simulink model "passive_new_wave_architecture_variable - Copy"  (R2021b)
settings: Solver=VariableStepAuto  StartTime=0.0  StopTime=20  RelTol=1e-5
values from neighbouring files (symbols this model uses):
  a1 = 1    [new_parameters.m]    (also in old.m; paper.m = 1.9; teleop_parameters_variable.m = 1.1)
  a2 = 1    [new_parameters.m]    (also in old.m; paper.m = 2.3; teleop_parameters_variable.m = 1.0101)
  b = 1    [new_parameters.m]    (also in old.m = 8.5; paper.m = 2.5; teleop_parameters_variable.m = 2.17; wave_s.m = block.InputPort(3).Data)
  B = 1.1    [new_parameters.m]    (also in obs_m.m = block.InputPort(4).Data; obs_s.m = block.InputPort(4).Data; old.m = 13; paper.m = 2)
  Be = 5    [new_parameters.m]    (also in old.m; paper.m; teleop_parameters_variable.m)
  beta = 1e-2    (= 0.01)    [new_parameters.m]    (also in old.m = 1.19e-07; paper.m = 2; teleop_parameters_variable.m = 0.0001)
  beta_m = 2*pi*Fc_vel*Ts    (= 0.0628318530718)    [new_parameters.m]    (also in old.m; paper.m; teleop_parameters_variable.m)
  beta_s = 2*pi*Fc_vel*Ts    (= 0.0628318530718)    [new_parameters.m]    (also in old.m; paper.m; teleop_parameters_variable.m)
  Bh = 0.02    [new_parameters.m]    (also in old.m; paper.m; teleop_parameters_variable.m)
  d_m2s = 1    [new_parameters.m]    (also in old.m = 2; paper.m = 2; teleop_parameters_variable.m = 2)
  delta = 1    [new_parameters.m]    (also in old.m; paper.m; teleop_parameters_variable.m = 100)
  eQ_m = 2*pi/4096    (= 0.00153398078789)    [new_parameters.m]    (also in old.m; paper.m; teleop_parameters_variable.m)
  eQ_s = 2*pi/4096    (= 0.00153398078789)    [new_parameters.m]    (also in old.m; paper.m; teleop_parameters_variable.m)
  Fc_h = 5    [new_parameters.m]    (also in old.m; paper.m; teleop_parameters_variable.m)
  Filter = 1    [old.m]
  Jh = 0.02    [new_parameters.m]    (also in old.m; paper.m; teleop_parameters_variable.m)
  k_m = 19.34    [new_parameters.m]    (also in old.m; paper.m; teleop_parameters_variable.m)
  k_s = 19.34    [new_parameters.m]    (also in old.m; paper.m; teleop_parameters_variable.m)
  ka = 0.001    [new_parameters.m]    (also in old.m = 0.0109; paper.m = 0.9; teleop_parameters_variable.m = 1)
  kb = 0.001    [new_parameters.m]    (also in old.m = 0.0089999; paper.m = 0.9; teleop_parameters_variable.m = 0.1)
  Kc2v_m = 4.5    [new_parameters.m]    (also in old.m; paper.m; teleop_parameters_variable.m)
  Kc2v_s = 4.5    [new_parameters.m]    (also in old.m; paper.m; teleop_parameters_variable.m)
  Kd_h = 0.5    [new_parameters.m]    (also in old.m; paper.m; teleop_parameters_variable.m)
  Kd_m = 0.5    [new_parameters.m]    (also in old.m; paper.m; teleop_parameters_variable.m)
  Kd_s = 0.5    [new_parameters.m]    (also in old.m; paper.m; teleop_parameters_variable.m)
  Ke = 10    [new_parameters.m]    (also in old.m; paper.m; teleop_parameters_variable.m = 100)
  Kp_h = 1.2    [new_parameters.m]    (also in old.m; paper.m; teleop_parameters_variable.m)
  Kp_m = 1    [new_parameters.m]    (also in old.m; paper.m; teleop_parameters_variable.m)
  Kp_s = 1    [new_parameters.m]    (also in old.m; paper.m; teleop_parameters_variable.m)
  Kt2c_m = 1.182    [new_parameters.m]    (also in old.m; paper.m; teleop_parameters_variable.m)
  Kt2c_s = 1.182    [new_parameters.m]    (also in old.m; paper.m; teleop_parameters_variable.m)
  lArm_m = 0.1    [new_parameters.m]    (also in old.m; paper.m; teleop_parameters_variable.m)
  lArm_s = 0.1    [new_parameters.m]    (also in old.m; paper.m; teleop_parameters_variable.m)
  M = 2    [new_parameters.m]    (also in obs_m.m = block.InputPort(5).Data; obs_s.m = block.InputPort(5).Data; old.m = 1; paper.m = 1)
  qe = 0.5    [new_parameters.m]    (also in old.m; paper.m; teleop_parameters_variable.m = 10)
  tau_m = 1.217    [new_parameters.m]    (also in old.m; paper.m; teleop_parameters_variable.m)
  tau_s = 1.217    [new_parameters.m]    (also in old.m; paper.m; teleop_parameters_variable.m)
  Ts = 0.001    [new_parameters.m]    (also in old.m; paper.m; teleop_parameters_variable.m)
libraries: simulink x2
settings Model: DataTypeOverride=Off  Creator=riccardo  LastModifiedBy=luigi
settings DebuggingCC: IgnoredZcDiagnostic=none  SFMachineParentedDataDiag=warning

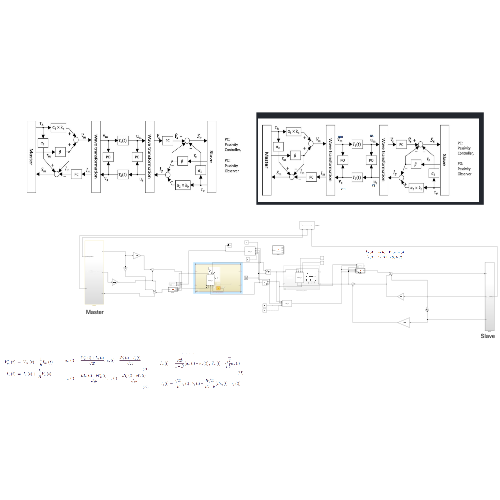
[thumbnail: Simulink's stored preview of the top-level diagram]
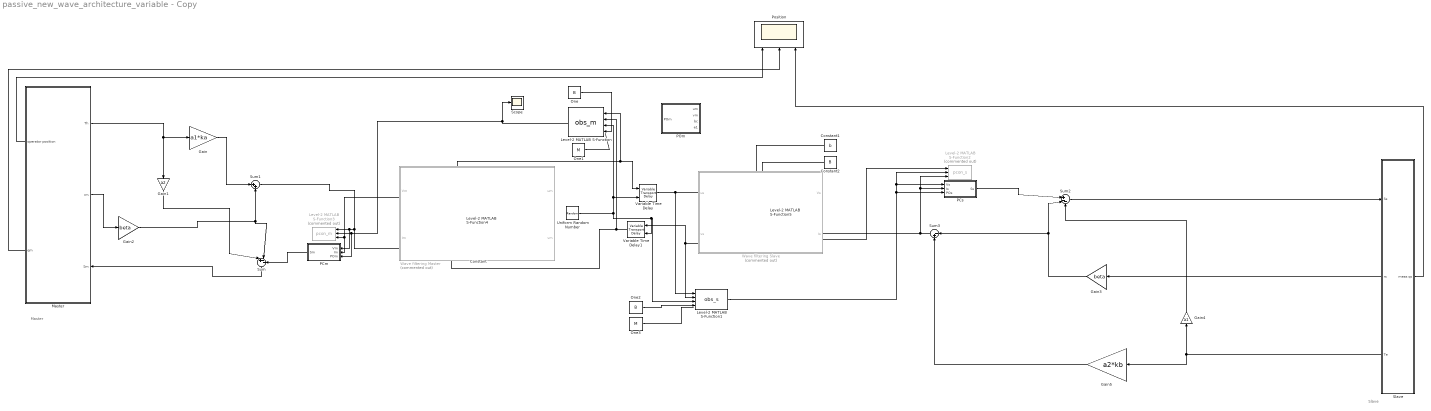
== system passive_new_wave_architecture_variable - Copy ==
  note: Slave
  note: Master
  Constant : Constant  Value=b
  Constant1 : Constant  Value=b
  Constant2 : Constant  Value=B
  Gain : Gain  Gain=a1*ka
  Gain1 : Gain  Gain=a2
  Gain2 : Gain  Gain=beta
  Gain3 : Gain  Gain=beta
  Gain4 : Gain  Gain=a1
  Gain5 : Gain  Gain=a2*kb
  Level-2 MATLAB S-Function : M-S-Function  FunctionName=obs_m
  Level-2 MATLAB S-Function1 : M-S-Function  FunctionName=obs_s
  Level-2 MATLAB S-Function2 : M-S-Function  Commented=on  FunctionName=pcon_s
  Level-2 MATLAB S-Function3 : M-S-Function  Commented=on  FunctionName=pcon_m
  Level-2 MATLAB S-Function4 : M-S-Function  FunctionName=wave_m
  Level-2 MATLAB S-Function5 : M-S-Function  FunctionName=wave_s
  Master : Subsystem
      settings: PortSchema="{\"entries\":[{\"content\":{\"sides\":[{\"content\":{\"connectorIds\":[\"Out3\",\"Out4\"]},\"type\":\"ConnectorPlacement.EquallySpacedRectSide\",\"uuid\":\"88a440f3-3c17-4ecd-8a7c-55e312326b6c\"},{\"content\":{\"connectorIds\":[\"Out1\",\"Out2\",\"In1\"],\"side\":\"RIGHT\"},\"type\":\"ConnectorPlacement.EquallySpacedRectSide\",\"uuid\":\"1f119ef7-309b-440c-9250-40a12b2cb029\"},{\"content\":{\"connectorIds\":[],\"side\":\"TOP\"},\"type\":\"ConnectorPlacement.EquallySpacedRectSide\",\"uuid\":\"7be3ae0e-cb45-4f37-96af-a21925a9e765\"}]},\"type\":\"ConnectorPlacement.EquallySpacedConnector\",\"uuid\":\"68cc326c-bdcb-4ff9-98f1-957be474a38c\"}],\"packageUris\":[\"http://schema.mathworks.com/mf0/Connector/R2020b\"],\"version\":\"1.0\"}"
  One : Constant  Value=B  OutDataTypeStr=Inherit: Inherit via back propagation
  One1 : Constant  Value=M  OutDataTypeStr=Inherit: Inherit via back propagation
  One2 : Constant  Value=B  OutDataTypeStr=Inherit: Inherit via back propagation
  One3 : Constant  Value=M  OutDataTypeStr=Inherit: Inherit via back propagation
  PCm : MATLAB Function  TreatAsAtomicUnit=on
  PCs : MATLAB Function  TreatAsAtomicUnit=on
  POm : MATLAB Function  TreatAsAtomicUnit=on
  Position : Scope  NumInputPorts=3
  Scope : Scope
  Slave : Subsystem
      settings: PortSchema="{\"entries\":[{\"content\":{\"sides\":[{\"content\":{\"connectorIds\":[\"In1\",\"Out2\",\"Out3\"]},\"type\":\"ConnectorPlacement.EquallySpacedRectSide\",\"uuid\":\"d7867d1a-8ca2-46eb-9cc5-3503a790e4da\"},{\"content\":{\"connectorIds\":[\"Out1\"],\"side\":\"RIGHT\"},\"type\":\"ConnectorPlacement.EquallySpacedRectSide\",\"uuid\":\"2f0413cf-eaaa-4002-929a-cebc19c82c9b\"},{\"content\":{\"connectorIds\":[],\"side\":\"TOP\"},\"type\":\"ConnectorPlacement.EquallySpacedRectSide\",\"uuid\":\"f97ed585-16ab-4e7f-97da-40ff87a224f1\"},{\"content\":{\"connectorIds\":[],\"side\":\"BOTTOM\"},\"type\":\"ConnectorPlacement.EquallySpacedRectSide\",\"uuid\":\"e911c9cd-6707-460b-adc0-d2ecc3cf8bb4\"}]},\"type\":\"ConnectorPlacement.EquallySpacedConnector\",\"uuid\":\"a99d57e5-6d89-49cd-b6f9-976c9398d117\"}],\"packageUris\":[\"http://schema.mathworks.com/mf0/Connector/R2020b\"],\"version\":\"1.0\"}"
  Sum : Sum  Inputs=|+--
  Sum1 : Sum  Inputs=|++
  Sum2 : Sum  Inputs=|+--
  Sum3 : Sum  Inputs=|-+
  Uniform Random Number : UniformRandomNumber  Minimum=0  Maximum=d_m2s  SampleTime=Ts  VectorParams1D=off
  Variable Time Delay : VariableTransportDelay  VariableDelayType=Variable transport delay  MaximumDelay=d_m2s  MaximumPoints=300000  ZeroDelay=on
  Variable Time Delay1 : VariableTransportDelay  VariableDelayType=Variable transport delay  MaximumDelay=d_s2m  MaximumPoints=300000  ZeroDelay=on
  Wave filtering Master : Subsystem  Commented=on
      settings: PortSchema="{\"entries\":[{\"content\":{\"sides\":[{\"content\":{\"connectorIds\":[\"In1\",\"Out2\"]},\"type\":\"ConnectorPlacement.EquallySpacedRectSide\",\"uuid\":\"022537ca-6b1a-446a-b70c-5cc8e9763a20\"},{\"content\":{\"connectorIds\":[\"Out1\",\"In2\"],\"side\":\"RIGHT\"},\"type\":\"ConnectorPlacement.EquallySpacedRectSide\",\"uuid\":\"d2fb6654-cfa2-4536-934e-f2f9b55519fe\"},{\"content\":{\"connectorIds\":[],\"side\":\"TOP\"},\"type\":\"ConnectorPlacement.EquallySpacedRectSide\",\"uuid\":\"40d1266d-c1ee-4ea7-83af-e87fd0883292\"}]},\"type\":\"ConnectorPlacement.EquallySpacedConnector\",\"uuid\":\"3d044237-6122-47a2-8c04-12fd83fac9c7\"}],\"packageUris\":[\"http://schema.mathworks.com/mf0/Connector/R2020b\"],\"version\":\"1.0\"}"
  Wave filtering Slave : Subsystem  Commented=on
      settings: PortSchema="{\"entries\":[{\"content\":{\"sides\":[{\"content\":{\"connectorIds\":[\"In1\",\"Out2\"]},\"type\":\"ConnectorPlacement.EquallySpacedRectSide\",\"uuid\":\"022537ca-6b1a-446a-b70c-5cc8e9763a20\"},{\"content\":{\"connectorIds\":[\"Out1\",\"In2\"],\"side\":\"RIGHT\"},\"type\":\"ConnectorPlacement.EquallySpacedRectSide\",\"uuid\":\"d2fb6654-cfa2-4536-934e-f2f9b55519fe\"},{\"content\":{\"connectorIds\":[],\"side\":\"TOP\"},\"type\":\"ConnectorPlacement.EquallySpacedRectSide\",\"uuid\":\"40d1266d-c1ee-4ea7-83af-e87fd0883292\"}]},\"type\":\"ConnectorPlacement.EquallySpacedConnector\",\"uuid\":\"3d044237-6122-47a2-8c04-12fd83fac9c7\"}],\"packageUris\":[\"http://schema.mathworks.com/mf0/Connector/R2020b\"],\"version\":\"1.0\"}"
  wires:
  Slave/1("meas qs ") -> Position/3
  Master/3("operator position ") -> Position/1
  Master/4(qm) -> Position/2
  Variable Time Delay1/1 -> Level-2 MATLAB S-Function4/2, Level-2 MATLAB S-Function/2
  Variable Time Delay/1 -> Level-2 MATLAB S-Function1/1, Level-2 MATLAB S-Function5/2
  Gain3/1 -> Sum2/2, Sum3/1
  Gain4/1 -> Sum2/3
  Sum3/1 -> Level-2 MATLAB S-Function2/3, PCs/2(Is), Level-2 MATLAB S-Function5/1
  Gain5/1 -> Sum3/2
  Sum2/1 -> Slave/1(Ss)
  Slave/2(rs) -> Gain3/1
  Sum/1 -> Master/1(Sm)
  Master/1(Th) -> Gain1/1, Gain/1
  Gain/1 -> Sum1/1
  Master/2(rm) -> Gain2/1
  Gain2/1 -> Sum/2, Sum1/2
  Gain1/1 -> Sum/1
  Uniform Random Number/1 -> Level-2 MATLAB S-Function/3, Variable Time Delay/2, Level-2 MATLAB S-Function1/3, Variable Time Delay1/2
  One1/1 -> ?
  One/1 -> Level-2 MATLAB S-Function/4
  One2/1 -> Level-2 MATLAB S-Function1/4
  One3/1 -> ?
  Slave/3(Te) -> Gain5/1, Gain4/1
  Level-2 MATLAB S-Function1/1 -> PCs/3(POs), PCs/1(Vs), Level-2 MATLAB S-Function2/2
  Level-2 MATLAB S-Function/1 -> Level-2 MATLAB S-Function3/2, PCm/3(POm), Scope/1
  Constant/1 -> Level-2 MATLAB S-Function4/3
  Sum1/1 -> PCm/1(Vm), Level-2 MATLAB S-Function3/1, Level-2 MATLAB S-Function4/1
  Level-2 MATLAB S-Function4/1 -> PCm/2(Im), Level-2 MATLAB S-Function3/3
  Level-2 MATLAB S-Function4/2 -> Level-2 MATLAB S-Function/1, Variable Time Delay/1
  Constant1/1 -> Level-2 MATLAB S-Function5/3
  Constant2/1 -> Level-2 MATLAB S-Function5/4
  Level-2 MATLAB S-Function5/1 -> Level-2 MATLAB S-Function2/1
  Level-2 MATLAB S-Function5/2 -> Variable Time Delay1/1, Level-2 MATLAB S-Function1/2
  PCm/1(Sm) -> Sum/3
  PCs/1(Ss) -> Sum2/1

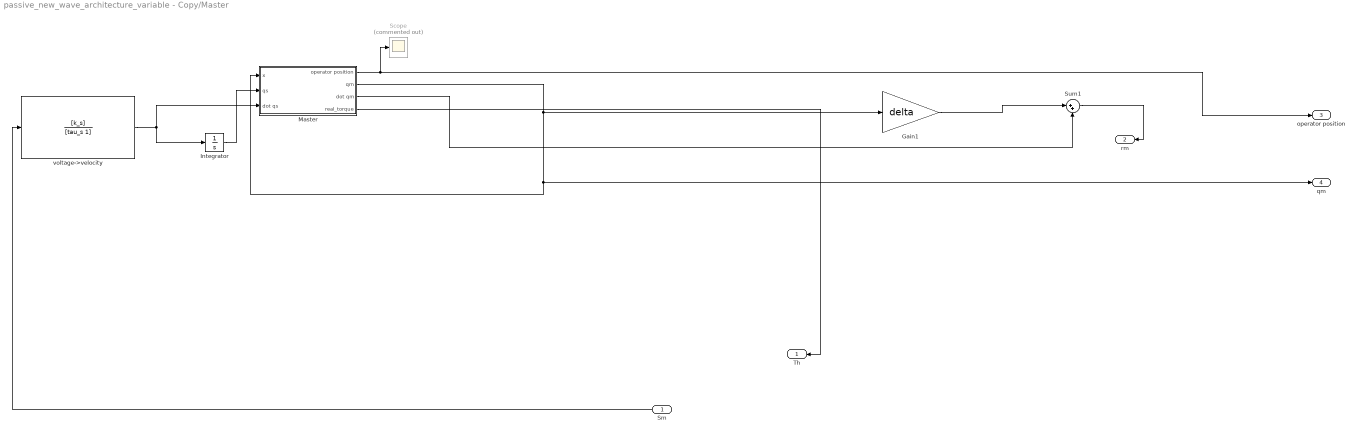
== system passive_new_wave_architecture_variable - Copy/Master ==
  Sm : Inport
  Gain1 : Gain  Gain=delta
  Integrator : Integrator
  Master : Subsystem
  Scope : Scope  Commented=on
  Sum1 : Sum  Inputs=|++
  voltage->velocity : TransferFcn  Numerator=[k_s]  Denominator=[tau_s 1]
  Th : Outport
  rm : Outport  Port=2
  "operator position " : Outport  Port=3
  qm : Outport  Port=4
  wires:
  Master/4(real_torque) -> Th/1
  voltage->velocity/1 -> Master/3(dot qs), Integrator/1
  Gain1/1 -> Sum1/1
  Integrator/1 -> Master/2(qs)
  Master/2(qm) -> Master/1(x), qm/1, Gain1/1
  Master/3(dot qm) -> Sum1/2
  Sm/1 -> voltage->velocity/1
  Master/1("operator position ") -> Scope/1, "operator position "/1
  Sum1/1 -> rm/1

== system passive_new_wave_architecture_variable - Copy/Slave ==
  Ss : Inport
  Gain : Gain  Gain=delta
  Integrator1 : Integrator
  Slave : Subsystem
  Sum : Sum  Inputs=|++
  voltage->velocity1 : TransferFcn  Numerator=[k_m]  Denominator=[tau_m 1]
  "meas qs " : Outport
  rs : Outport  Port=2
  Te : Outport  Port=3
  wires:
  Sum/1 -> rs/1
  Slave/1("meas qs ") -> "meas qs "/1, Gain/1
  Slave/3(slave torque) -> Te/1
  Gain/1 -> Sum/1
  Slave/2("Vel Stimata ") -> Sum/2
  voltage->velocity1/1 -> Integrator1/1, Slave/2(dot_xd)
  Ss/1 -> voltage->velocity1/1
  Integrator1/1 -> Slave/1(xd)

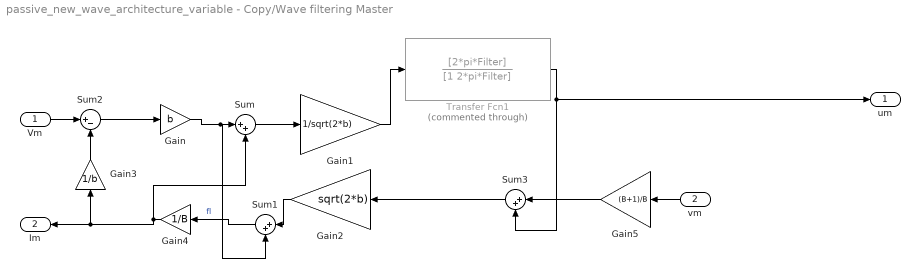
== system passive_new_wave_architecture_variable - Copy/Wave filtering Master ==
  Vm : Inport
  vm : Inport  Port=2
  Gain : Gain  Gain=b
  Gain1 : Gain  Gain=1/sqrt(2*b)
  Gain2 : Gain  Gain=sqrt(2*b)
  Gain3 : Gain  Gain=1/b
  Gain4 : Gain  Gain=1/B
  Gain5 : Gain  Gain=(B+1)/B
  Sum : Sum  Inputs=|++
  Sum1 : Sum  Inputs=|++
  Sum2 : Sum  Inputs=|+-
  Sum3 : Sum  Inputs=|++
  Transfer Fcn1 : TransferFcn  Commented=through  Numerator=[2*pi*Filter]  Denominator=[1 2*pi*Filter]
  um : Outport
  Im : Outport  Port=2
  wires:
  Gain/1 -> Sum1/2, Sum/1
  Sum/1 -> Gain1/1
  Gain2/1 -> Sum1/1
  Sum1/1 -> Gain4/1  "fl"
  Vm/1 -> Sum2/1
  Sum2/1 -> Gain/1
  Gain3/1 -> Sum2/2
  Gain4/1 -> Im/1, Gain3/1, Sum/2
  vm/1 -> Gain5/1
  Sum3/1 -> Gain2/1
  Gain5/1 -> Sum3/1
  Gain1/1 -> Transfer Fcn1/1
  Transfer Fcn1/1 -> um/1, Sum3/2

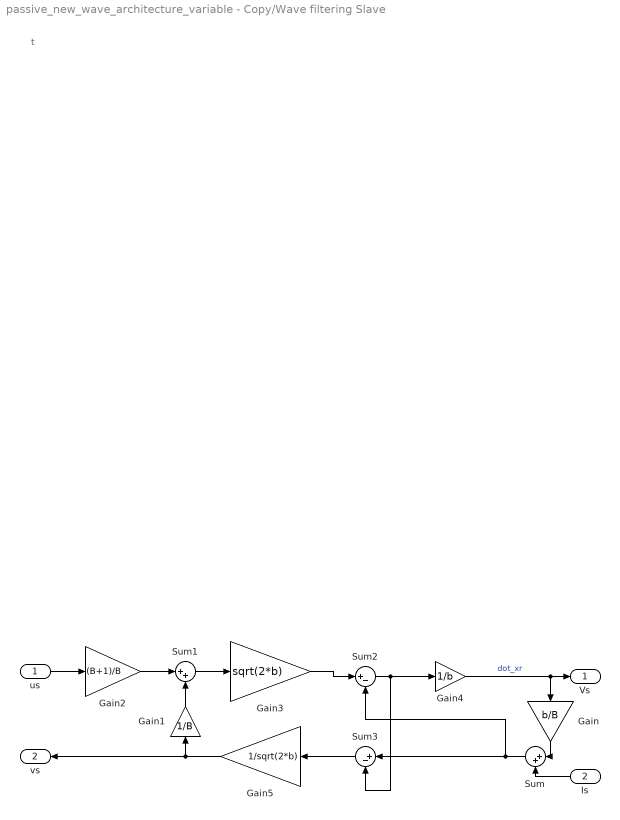
== system passive_new_wave_architecture_variable - Copy/Wave filtering Slave ==
  note: t
  us : Inport
  Is : Inport  Port=2
  Gain : Gain  Gain=b/B
  Gain1 : Gain  Gain=1/B
  Gain2 : Gain  Gain=(B+1)/B
  Gain3 : Gain  Gain=sqrt(2*b)
  Gain4 : Gain  Gain=1/b
  Gain5 : Gain  Gain=1/sqrt(2*b)
  Sum : Sum  Inputs=|++
  Sum1 : Sum  Inputs=|++
  Sum2 : Sum  Inputs=|+-
  Sum3 : Sum  Inputs=|+-
  Vs : Outport
  vs : Outport  Port=2
  wires:
  Sum2/1 -> Sum3/2, Gain4/1
  Gain3/1 -> Sum2/1
  Sum3/1 -> Gain5/1
  Gain4/1 -> Gain/1, Vs/1  "dot_xr"
  Gain5/1 -> Gain1/1, vs/1
  Sum/1 -> Sum2/2, Sum3/1
  Is/1 -> Sum/2
  Gain/1 -> Sum/1
  Gain1/1 -> Sum1/2
  us/1 -> Gain2/1
  Sum1/1 -> Gain3/1
  Gain2/1 -> Sum1/1

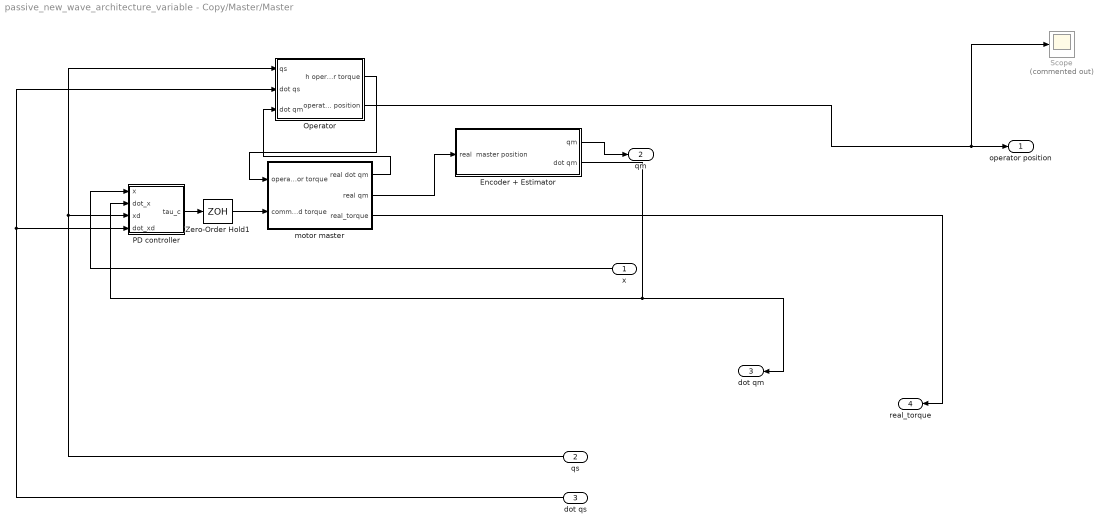
== system passive_new_wave_architecture_variable - Copy/Master/Master ==
  x : Inport
  qs : Inport  Port=2
  dot qs : Inport  Port=3
  Encoder + Estimator : Subsystem
  Operator : Subsystem
  PD controller : Subsystem
  Scope : Scope  Commented=on
  Zero-Order Hold1 : ZeroOrderHold  SampleTime=Ts
  motor master : Subsystem
  "operator position " : Outport
  qm : Outport  Port=2
  dot qm : Outport  Port=3
  real_torque : Outport  Port=4
  wires:
  motor master/1(real dot qm) -> Operator/3(dot qm)
  PD controller/1(tau_c) -> Zero-Order Hold1/1
  qs/1 -> Operator/1(qs), PD controller/3(xd)
  motor master/2(real qm) -> Encoder + Estimator/1(real  master position)
  Operator/1(h operator torque) -> motor master/1(operator torque)
  dot qs/1 -> Operator/2(dot qs), PD controller/4(dot_xd)
  Encoder + Estimator/2(dot qm) -> dot qm/1, PD controller/2(dot_x)
  Encoder + Estimator/1(qm) -> qm/1
  Zero-Order Hold1/1 -> motor master/2(command torque)
  motor master/3(real_torque) -> real_torque/1
  Operator/2("operator position ") -> Scope/1, "operator position "/1
  x/1 -> PD controller/1(x)

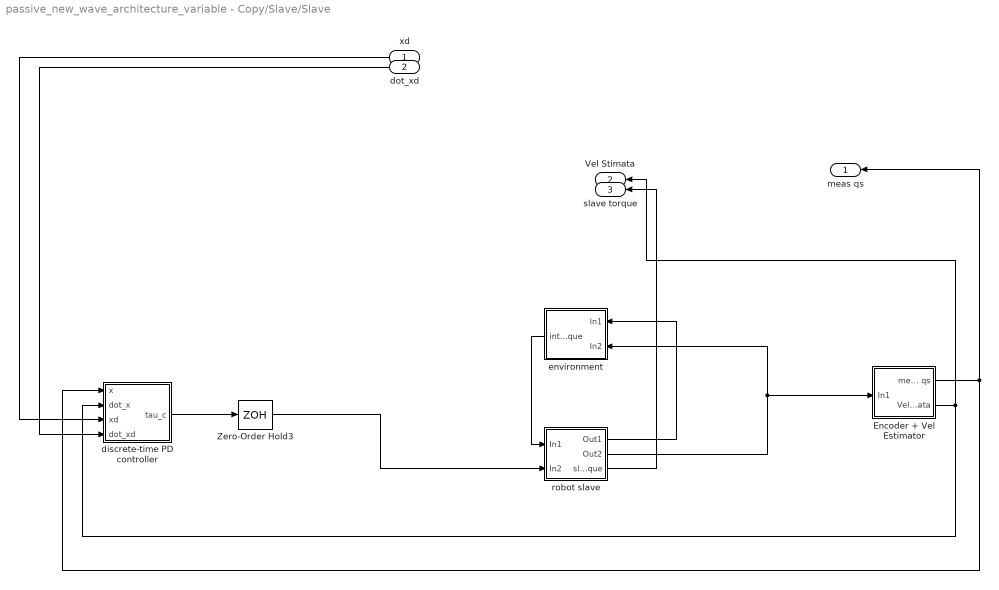
== system passive_new_wave_architecture_variable - Copy/Slave/Slave ==
  xd : Inport
  dot_xd : Inport  Port=2
  "Encoder + Vel Estimator " : Subsystem
  Zero-Order Hold3 : ZeroOrderHold  SampleTime=Ts
  discrete-time PD controller : Subsystem
  "environment " : Subsystem
  "robot slave " : Subsystem
  "meas qs " : Outport
  "Vel Stimata " : Outport  Port=2
  slave torque : Outport  Port=3
  wires:
  "robot slave "/1(Out1) -> "environment "/1(In1)
  "robot slave "/2(Out2) -> "environment "/2(In2), "Encoder + Vel Estimator "/1(In1)
  "Encoder + Vel Estimator "/1("meas qs ") -> "meas qs "/1, discrete-time PD controller/1(x)
  Zero-Order Hold3/1 -> "robot slave "/2(In2)
  "Encoder + Vel Estimator "/2("Vel Stimata ") -> "Vel Stimata "/1, discrete-time PD controller/2(dot_x)
  discrete-time PD controller/1(tau_c) -> Zero-Order Hold3/1
  "environment "/1("interaction torque ") -> "robot slave "/1(In1)
  dot_xd/1 -> discrete-time PD controller/4(dot_xd)
  xd/1 -> discrete-time PD controller/3(xd)
  "robot slave "/3(slave torque) -> slave torque/1

== system passive_new_wave_architecture_variable - Copy/Master/Master/Encoder + Estimator ==
  real  master position : Inport
  Constant : Constant  Value=eQ_m
  Sum : Sum  Inputs=++|
  Velocity estimator : Subsystem
  Zero-Order Hold : ZeroOrderHold  SampleTime=Ts
  noise : MATLAB Function  TreatAsAtomicUnit=on
  qm : Outport
  dot qm : Outport  Port=2
  wires:
  real  master position/1 -> Zero-Order Hold/1
  Zero-Order Hold/1 -> Sum/2
  Sum/1 -> qm/1, Velocity estimator/1(pos misurata)
  Constant/1 -> noise/1(delta_q)
  Velocity estimator/1(Vel stimata) -> dot qm/1
  noise/1(error) -> Sum/1

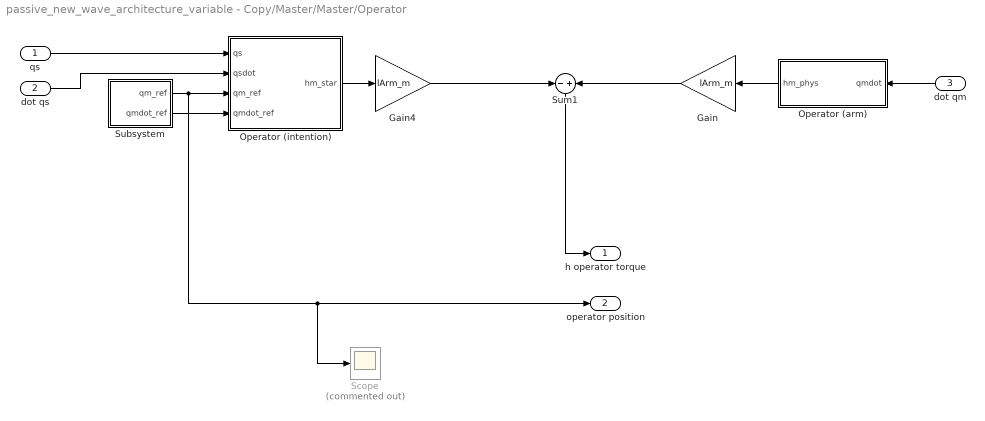
== system passive_new_wave_architecture_variable - Copy/Master/Master/Operator ==
  qs : Inport
  dot qs : Inport  Port=2
  dot qm : Inport  Port=3
  Gain : Gain  Gain=lArm_m
  Gain4 : Gain  Gain=lArm_m
  Operator (arm) : Subsystem
  Operator (intention) : Subsystem
  Scope : Scope  Commented=on
  Subsystem : Subsystem
  Sum1 : Sum  Inputs=-+
  h operator torque : Outport
  "operator position " : Outport  Port=2
  wires:
  Sum1/1 -> h operator torque/1
  Operator (arm)/1(hm_phys) -> Gain/1
  dot qm/1 -> Operator (arm)/1(qmdot)
  Subsystem/2(qmdot_ref) -> Operator (intention)/4(qmdot_ref)
  Operator (intention)/1(hm_star) -> Gain4/1
  dot qs/1 -> Operator (intention)/2(qsdot)
  Gain4/1 -> Sum1/1
  Gain/1 -> Sum1/2
  Subsystem/1(qm_ref) -> Scope/1, "operator position "/1, Operator (intention)/3(qm_ref)
  qs/1 -> Operator (intention)/1(qs)

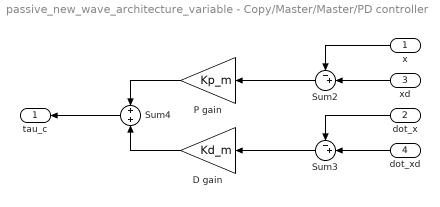
== system passive_new_wave_architecture_variable - Copy/Master/Master/PD controller ==
  x : Inport
  dot_x : Inport  Port=2
  xd : Inport  Port=3
  dot_xd : Inport  Port=4
  D gain : Gain  Gain=Kd_m
  P gain : Gain  Gain=Kp_m
  Sum2 : Sum  Inputs=-+|
  Sum3 : Sum  Inputs=-+|
  Sum4 : Sum
  tau_c : Outport  VectorParamsAs1DForOutWhenUnconnected=off
  wires:
  D gain/1 -> Sum4/2
  dot_x/1 -> Sum3/1
  dot_xd/1 -> Sum3/2
  x/1 -> Sum2/1
  xd/1 -> Sum2/2
  Sum3/1 -> D gain/1
  P gain/1 -> Sum4/1
  Sum4/1 -> tau_c/1
  Sum2/1 -> P gain/1

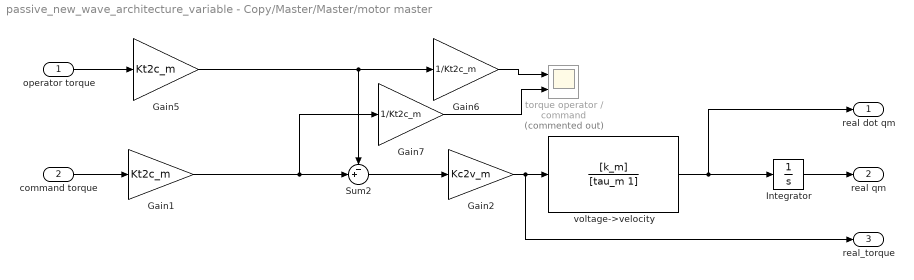
== system passive_new_wave_architecture_variable - Copy/Master/Master/motor master ==
  operator torque : Inport
  command torque : Inport  Port=2
  Gain1 : Gain  Gain=Kt2c_m
  Gain2 : Gain  Gain=Kc2v_m
  Gain5 : Gain  Gain=Kt2c_m
  Gain6 : Gain  Gain=1/Kt2c_m
  Gain7 : Gain  Gain=1/Kt2c_m
  Integrator : Integrator
  Sum2 : Sum  Inputs=-+|
  torque operator / command : Scope  Commented=on  NumInputPorts=2
  voltage->velocity : TransferFcn  Numerator=[k_m]  Denominator=[tau_m 1]
  real dot qm : Outport
  real qm : Outport  Port=2
  real_torque : Outport  Port=3
  wires:
  Gain7/1 -> torque operator / command/2
  operator torque/1 -> Gain5/1
  Gain2/1 -> real_torque/1, voltage->velocity/1
  Gain1/1 -> Gain7/1, Sum2/2
  Integrator/1 -> real qm/1
  command torque/1 -> Gain1/1
  Gain6/1 -> torque operator / command/1
  voltage->velocity/1 -> real dot qm/1, Integrator/1
  Sum2/1 -> Gain2/1
  Gain5/1 -> Sum2/1, Gain6/1

== system passive_new_wave_architecture_variable - Copy/Slave/Slave/Encoder + Vel Estimator  ==
  In1 : Inport
  Constant : Constant  Value=eQ_s
  Subsystem : Subsystem
  Sum : Sum  Inputs=++|
  Zero-Order Hold : ZeroOrderHold  SampleTime=Ts
  noise : MATLAB Function  TreatAsAtomicUnit=on
  "meas qs " : Outport
  "Vel Stimata " : Outport  Port=2
  wires:
  Constant/1 -> noise/1(delta_q)
  In1/1 -> Zero-Order Hold/1
  noise/1(error) -> Sum/1
  Zero-Order Hold/1 -> Sum/2
  Sum/1 -> "meas qs "/1, Subsystem/1(pos misurata)
  Subsystem/1(Vel stimata) -> "Vel Stimata "/1

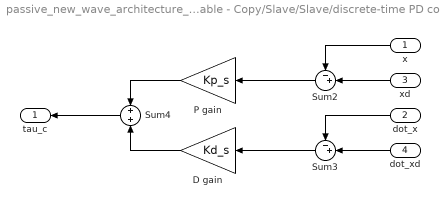
== system passive_new_wave_architecture_variable - Copy/Slave/Slave/discrete-time PD controller ==
  x : Inport
  dot_x : Inport  Port=2
  xd : Inport  Port=3
  dot_xd : Inport  Port=4
  D gain : Gain  Gain=Kd_s
  P gain : Gain  Gain=Kp_s
  Sum2 : Sum  Inputs=-+|
  Sum3 : Sum  Inputs=-+|
  Sum4 : Sum
  tau_c : Outport  VectorParamsAs1DForOutWhenUnconnected=off
  wires:
  D gain/1 -> Sum4/2
  dot_x/1 -> Sum3/1
  dot_xd/1 -> Sum3/2
  x/1 -> Sum2/1
  xd/1 -> Sum2/2
  Sum3/1 -> D gain/1
  P gain/1 -> Sum4/1
  Sum4/1 -> tau_c/1
  Sum2/1 -> P gain/1

== system passive_new_wave_architecture_variable - Copy/Slave/Slave/environment  ==
  note: qs
  note: qdot
  In1 : Inport
  In2 : Inport  Port=2
  Environment : Subsystem
  Gain : Gain  Gain=lArm_s
  "interaction torque " : Outport
  wires:
  In2/1 -> Environment/2(qs)
  Environment/1(fe) -> Gain/1
  In1/1 -> Environment/1(qsdot)
  Gain/1 -> "interaction torque "/1

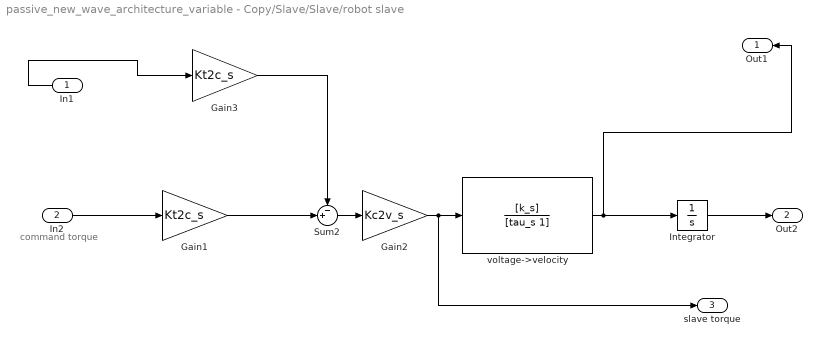
== system passive_new_wave_architecture_variable - Copy/Slave/Slave/robot slave  ==
  note: command torque
  In1 : Inport
  In2 : Inport  Port=2
  Gain1 : Gain  Gain=Kt2c_s
  Gain2 : Gain  Gain=Kc2v_s
  Gain3 : Gain  Gain=Kt2c_s
  Integrator : Integrator
  Sum2 : Sum  Inputs=-+|
  voltage->velocity : TransferFcn  Numerator=[k_s]  Denominator=[tau_s 1]
  Out1 : Outport
  Out2 : Outport  Port=2
  slave torque : Outport  Port=3
  wires:
  Gain2/1 -> slave torque/1, voltage->velocity/1
  Gain3/1 -> Sum2/1
  voltage->velocity/1 -> Out1/1, Integrator/1
  Gain1/1 -> Sum2/2
  Sum2/1 -> Gain2/1
  Integrator/1 -> Out2/1
  In1/1 -> Gain3/1
  In2/1 -> Gain1/1

== system passive_new_wave_architecture_variable - Copy/Master/Master/Encoder + Estimator/Velocity estimator ==
  pos misurata : Inport
  Difference : simulink/Discrete/Difference  ICPrevInput=0.0  OutMin=[]  OutMax=[]  OutDataType=fixdt(1, 16)  OutScaling=2^-10  DoSatur=off
  Filtro passabasso : DiscreteTransferFcn  Numerator=[beta_m 0]  Denominator=[1 -(1-beta_m)]  SampleTime=Ts
  Gain2 : Gain  Gain=1/Ts
  Vel stimata : Outport  VectorParamsAs1DForOutWhenUnconnected=off
  wires:
  Gain2/1 -> Filtro passabasso/1
  pos misurata/1 -> Difference/1
  Difference/1 -> Gain2/1
  Filtro passabasso/1 -> Vel stimata/1  "Velocità  stimata"

== system passive_new_wave_architecture_variable - Copy/Master/Master/Operator/Operator (arm) ==
  note: force
  qmdot : Inport
  Derivative : Derivative  CoefficientInTFapproximation=0.001
  Gain1 : Gain  Gain=Jh
  Gain2 : Gain  Gain=Bh
  Sum : Sum  Inputs=+|+
  hm_phys : Outport  VectorParamsAs1DForOutWhenUnconnected=off
  wires:
  qmdot/1 -> Gain2/1, Derivative/1
  Sum/1 -> hm_phys/1
  Derivative/1 -> Gain1/1
  Gain2/1 -> Sum/1
  Gain1/1 -> Sum/2

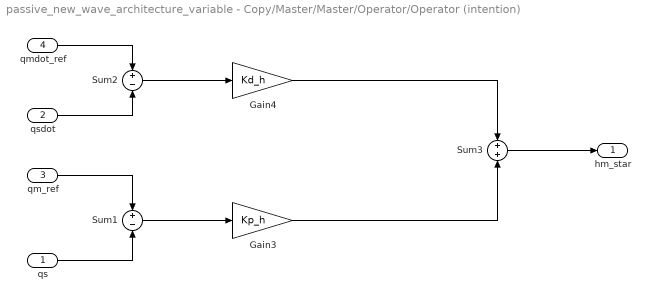
== system passive_new_wave_architecture_variable - Copy/Master/Master/Operator/Operator (intention) ==
  qs : Inport
  qsdot : Inport  Port=2
  qm_ref : Inport  Port=3
  qmdot_ref : Inport  Port=4
  Gain3 : Gain  Gain=Kp_h
  Gain4 : Gain  Gain=Kd_h
  Sum1 : Sum  Inputs=+|-
  Sum2 : Sum  Inputs=+|-
  Sum3 : Sum  Inputs=+|+
  hm_star : Outport  VectorParamsAs1DForOutWhenUnconnected=off
  wires:
  qs/1 -> Sum1/2
  qm_ref/1 -> Sum1/1
  qmdot_ref/1 -> Sum2/1
  Sum1/1 -> Gain3/1
  qsdot/1 -> Sum2/2
  Sum2/1 -> Gain4/1
  Gain4/1 -> Sum3/1
  Gain3/1 -> Sum3/2
  Sum3/1 -> hm_star/1

== system passive_new_wave_architecture_variable - Copy/Master/Master/Operator/Subsystem ==
  Derivative1 : Derivative  CoefficientInTFapproximation=0.001
  Manual Switch : ManualSwitch  CurrentSetting=0
  Sine Wave : Sin  SampleTime=0
  Step : Step  SampleTime=0
  low-pass filter : TransferFcn  Numerator=[2*pi*Fc_h]  Denominator=[1 2*pi*Fc_h]
  qm_ref : Outport
  qmdot_ref : Outport  Port=2
  wires:
  low-pass filter/1 -> Manual Switch/2
  Manual Switch/1 -> qm_ref/1, Derivative1/1
  Derivative1/1 -> qmdot_ref/1  "qmdot_ref"
  Step/1 -> low-pass filter/1
  Sine Wave/1 -> Manual Switch/1

== system passive_new_wave_architecture_variable - Copy/Slave/Slave/Encoder + Vel Estimator /Subsystem ==
  pos misurata : Inport
  Difference : simulink/Discrete/Difference  ICPrevInput=0.0  OutMin=[]  OutMax=[]  OutDataType=fixdt(1, 16)  OutScaling=2^-10  DoSatur=off
  Filtro passabasso : DiscreteTransferFcn  Numerator=[beta_s 0]  Denominator=[1 -(1-beta_s)]  SampleTime=Ts
  Gain2 : Gain  Gain=1/Ts
  Vel stimata : Outport  VectorParamsAs1DForOutWhenUnconnected=off
  wires:
  Gain2/1 -> Filtro passabasso/1
  pos misurata/1 -> Difference/1
  Difference/1 -> Gain2/1
  Filtro passabasso/1 -> Vel stimata/1  "Velocità  stimata"

== system passive_new_wave_architecture_variable - Copy/Slave/Slave/environment /Environment ==
  note: force
  qsdot : Inport
  qs : Inport  Port=2
  Constant : Constant  Value=qe  SampleTime=0
  c1 : Constant  Value=Be  SampleTime=0
  c2 : Constant  Value=Ke  SampleTime=0
  env : MATLAB Function  TreatAsAtomicUnit=on
  fe : Outport  VectorParamsAs1DForOutWhenUnconnected=off
  wires:
  Constant/1 -> env/3(qe)
  c1/1 -> env/2(Be)
  c2/1 -> env/1(Ke)
  qs/1 -> env/4(qs)
  qsdot/1 -> env/5(qsdot)
  env/1(fE) -> fe/1

== matlab function passive_new_wave_architecture_variable - Copy/Slave/Slave/Encoder + Vel Estimator /noise ==
  data: delta_q input; error output
function error = noise_measurement(delta_q)
if randn(1)>0
   error = delta_q;
else
    error = -delta_q;
end

== matlab function passive_new_wave_architecture_variable - Copy/Master/Master/Encoder + Estimator/noise ==
  data: delta_q input; error output
function error = noise_measurement(delta_q)
if randn(1)>0
   error = delta_q;
else
    error = -delta_q;
end

== matlab function passive_new_wave_architecture_variable - Copy/PCs ==
  data: Vs input; Is input; POs input; Ss output
function Ss  = pcon_s(Vs,Is,POs)
  if POs > 0
      L2=0;
  elseif (Is*Is)>0
      L2=-POs/(Is*Is);
  else
      L2=0;
  end

  Ss = Vs + L2*Is;

== matlab function passive_new_wave_architecture_variable - Copy/PCm ==
  data: Vm input; Im input; POm input; Sm output
function Sm  = pcon_m(Vm,Im,POm)
  if POm > 0
      L1=0;
  elseif (Vm*Vm)>0
      L1=-POm/(Vm*Vm);
  else
      L1=0;
  end
  
  Sm = Im + L1*Vm;

== matlab function passive_new_wave_architecture_variable - Copy/POm ==
  data: um input; vm input; bc input; POm output; e1 input
function POm  = pobs_m(um,vm,bc,e1)
    Tm=um;
    qm=vm;
    b=bc;
    POm = (1/b)*Tm*Tm - (1/(2*b))*((Tm-b*qm)*(Tm-b*qm)) - (1/(2*b))*e1*Tm*Tm;

== matlab function passive_new_wave_architecture_variable - Copy/Slave/Slave/environment /Environment/env ==
  data: Ke input; Be input; qe input; qs input; fE output; qsdot input
function fE  = environment(Ke, Be, qe, qs, qsdot)
if qs > qe
   fE = Ke * (qs - qe);%+ Be * qsdot;
else
   fE = 0;
end
